simulink library "tether2node_ul"  (R2018b)
settings: Solver=VariableStepAuto  StartTime=0.0  StopTime=10.0  RelTol=1e-3
undefined symbols (not defined in the file or in its folder): massBdy, N, numNode, rhoFluid
libraries: tetherDragForce_ul x1, tetherInternalForces_ul x1
settings Model: Creator=asiddiq2  LastModifiedBy=asiddiq2

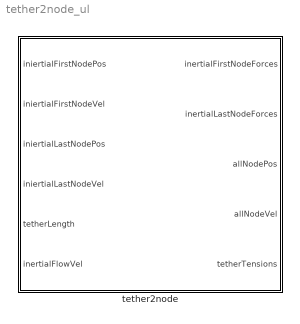
== system tether2node_ul ==
  tether2node : Subsystem  mask{rhoFluid=rhoFluid, massBdy=massBdy, numNode=numNode, thrDia=0, thrRho=0, thrYoungs=0, thrZeta=0, thrCd=0}
      mask prompts: rhoFluid "Fluid density"; massBdy "Vehicle Mass (kg)"; numNode "Number of Nodes"; thrDia "Tether diameter"; thrRho "Tether density"; thrYoungs "Tether Youngs modulus"; thrZeta "Tether damping ratio"; thrCd "Tether drag coefficient"
      mask TypeOptions rhoFluid: tetherNodalDragForces/rhoFluid
      mask TypeOptions massBdy: tetherNodalinternalForces/massBdy
      mask TypeOptions numNode: tetherNodalDragForces/numNode | tetherNodalinternalForces/numNode
      mask DialogControl ParameterGroupVar Prompt: Environment
      mask DialogControl Container3 Prompt: Vehicle
      mask DialogControl Container4 Prompt: Tether

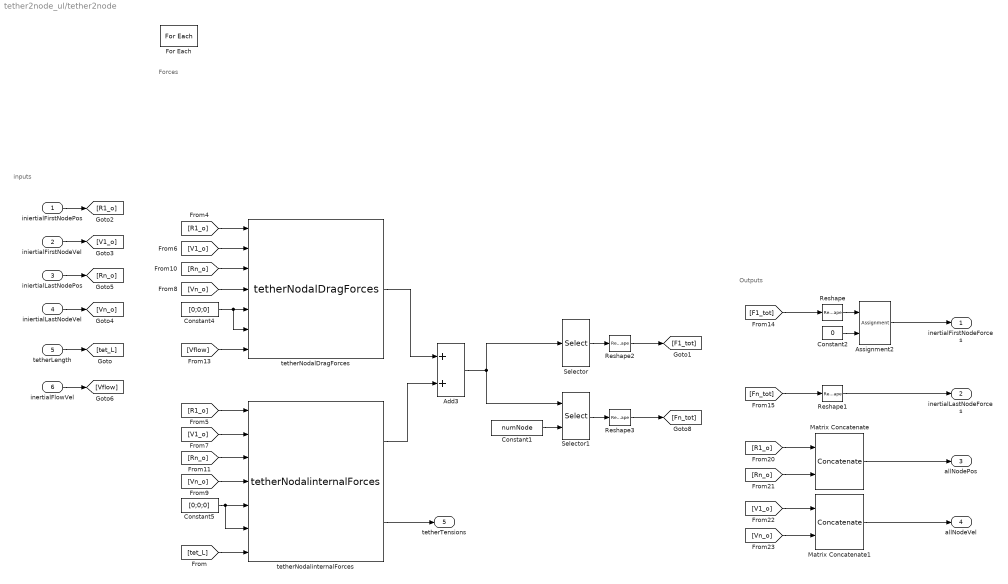
== system tether2node_ul/tether2node ==
  note: inputs
  note: Outputs
  note: Forces
  iniertialFirstNodePos : Inport  PortDimensions=[3,1]  Partition=on  PartitionDimension=2  PartitionWidth=1  PartitionOffset=0
  iniertialFirstNodeVel : Inport  Port=2  PortDimensions=[3,1]  Partition=on  PartitionDimension=2  PartitionWidth=1  PartitionOffset=0
  iniertialLastNodePos : Inport  Port=3  PortDimensions=[3,1]  Partition=on  PartitionDimension=2  PartitionWidth=1  PartitionOffset=0
  iniertialLastNodeVel : Inport  Port=4  PortDimensions=[3,1]  Partition=on  PartitionDimension=2  PartitionWidth=1  PartitionOffset=0
  tetherLength : Inport  Port=5  PortDimensions=[1,1]  Partition=on  PartitionDimension=2  PartitionWidth=1  PartitionOffset=0
  inertialFlowVel : Inport  Port=6  PortDimensions=[3,1]
  Add3 : Sum
  Assignment2 : Assignment  NumberOfDimensions=2  DiagnosticForDimensions=Warning  IndexOptions=Index vector (dialog),Index vector (dialog)  Indices=3,1  OutputSizes=1,1
  Constant1 : Constant  Value=numNode  VectorParams1D=off
  Constant2 : Constant  Value=0
  Constant4 : Constant  Value=[0;0;0]  VectorParams1D=off
  Constant5 : Constant  Value=[0;0;0]  VectorParams1D=off
  For Each : ForEach  DisableCoverage=on  IterateSubsysMaskParameter=off,off,off,on,on,on,on,on  SubsysMaskParameterIterationDimension=1,1,1,2,2,2,2,2  IndexMode=One-based
  Matrix Concatenate : Concatenate  Mode=Multidimensional array  ConcatenateDimension=2
  Matrix Concatenate1 : Concatenate  Mode=Multidimensional array  ConcatenateDimension=2
  Reshape{,1..3} (4 alike) : Reshape  OutputDimensionality=Column vector (2-D)
  Selector : Selector  NumberOfDimensions=2  InputPortWidth=3  IndexOptions=Select all,Index vector (dialog)  Indices=[1 3],1  OutputSizes=1,1
  Selector1 : Selector  NumberOfDimensions=2  InputPortWidth=3  IndexOptions=Select all,Index vector (port)  Indices=[1 3],N  OutputSizes=1,1
  tetherNodalDragForces : tetherDragForce_ul/tetherNodalDragForces  rhoFluid=rhoFluid  numNode=numNode  diaTether=thrDia  CdTether=thrCd
  tetherNodalinternalForces : tetherInternalForces_ul/tetherNodalinternalForces  massBdy=massBdy  numNode=numNode  diaTether=thrDia  youngsTether=thrYoungs  zetaTether=thrZeta
  inertialFirstNodeForces : Outport  PortDimensions=[3,1]  ConcatenationDimension=2
  inertialLastNodeForces : Outport  Port=2  PortDimensions=[3,1]  ConcatenationDimension=2
  allNodePos : Outport  Port=3  PortDimensions=[3,numNode]  ConcatenationDimension=3
  allNodeVel : Outport  Port=4  PortDimensions=[3,numNode]  ConcatenationDimension=3
  tetherTensions : Outport  Port=5  ConcatenationDimension=3
  wires:
  [Vn_o] -> tetherNodalinternalForces/4
  inertialFlowVel/1 -> [Vflow]
  tetherNodalDragForces/1 -> Add3/1
  Constant5/1 -> tetherNodalinternalForces/6, tetherNodalinternalForces/5
  Selector/1 -> Reshape2/1
  iniertialFirstNodePos/1 -> [R1_o]
  [Vn_o] -> tetherNodalDragForces/4
  Matrix Concatenate1/1 -> allNodeVel/1
  Add3/1 -> Selector/1, Selector1/1
  tetherLength/1 -> [tet_L]
  Selector1/1 -> Reshape3/1
  [Rn_o] -> Matrix Concatenate/2
  [Rn_o] -> tetherNodalDragForces/3
  [F1_tot] -> Reshape/1
  Reshape1/1 -> inertialLastNodeForces/1
  [R1_o] -> tetherNodalDragForces/1
  iniertialLastNodePos/1 -> [Rn_o]
  [Vflow] -> tetherNodalDragForces/7
  Matrix Concatenate/1 -> allNodePos/1
  Reshape3/1 -> [Fn_tot]
  iniertialFirstNodeVel/1 -> [V1_o]
  Constant1/1 -> Selector1/2
  [Fn_tot] -> Reshape1/1
  Reshape2/1 -> [F1_tot]
  [V1_o] -> tetherNodalinternalForces/2
  Reshape/1 -> Assignment2/1
  [V1_o] -> Matrix Concatenate1/1
  [V1_o] -> tetherNodalDragForces/2
  Constant4/1 -> tetherNodalDragForces/6, tetherNodalDragForces/5
  tetherNodalinternalForces/1 -> Add3/2
  [Vn_o] -> Matrix Concatenate1/2
  tetherNodalinternalForces/2 -> tetherTensions/1
  [R1_o] -> tetherNodalinternalForces/1
  [R1_o] -> Matrix Concatenate/1
  [tet_L] -> tetherNodalinternalForces/7
  iniertialLastNodeVel/1 -> [Vn_o]
  [Rn_o] -> tetherNodalinternalForces/3
  Assignment2/1 -> inertialFirstNodeForces/1
  Constant2/1 -> Assignment2/2
